simulink model "NoVCU"  (R2025b)
settings: configuration reference "VehicleFixed10ms" (kept outside this file)
undefined symbols (not defined in the file): PlntEngTqMax
settings Model: DataDictionary=VirtualMotoTemplate.sldd  ModifiedByFormat=The MathWorks, Inc.  Creator=The MathWorks, Inc.  LastModifiedBy=The MathWorks, Inc.
settings ConfigSetRef: SourceName=VehicleFixed10ms

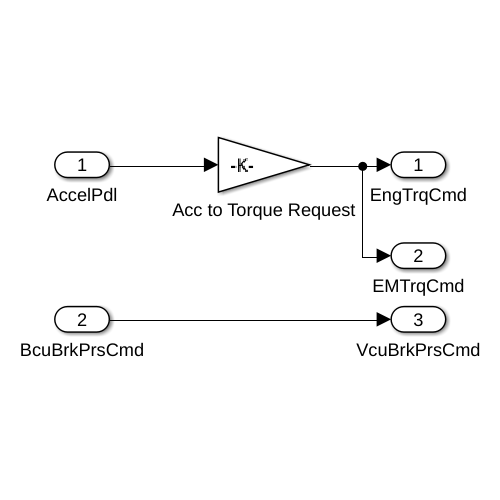
[thumbnail: Simulink's stored preview of the top-level diagram]
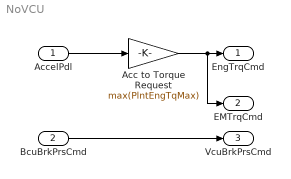
== system NoVCU ==
  AccelPdl : Inport
  BcuBrkPrsCmd : Inport  Port=2  SampleTime=0.01
  Acc to Torque Request : Gain  Gain=max(PlntEngTqMax)
  EngTrqCmd : Outport  OutDataTypeStr=double  PortDimensions=1  SampleTime=[0.01,0]  VectorParamsAs1DForOutWhenUnconnected=off
  EMTrqCmd : Outport  Port=2  VectorParamsAs1DForOutWhenUnconnected=off
  VcuBrkPrsCmd : Outport  Port=3  PortDimensions=2  VectorParamsAs1DForOutWhenUnconnected=off
  wires:
  Acc to Torque Request/1 -> EMTrqCmd/1, EngTrqCmd/1
  BcuBrkPrsCmd/1 -> VcuBrkPrsCmd/1
  AccelPdl/1 -> Acc to Torque Request/1
